simulink model "ProblemStatement1_Modulation"  (R2021a)
settings: Solver=VariableStepAuto  StartTime=0.0  StopTime=10.0  RelTol=1e-3
settings Model: Creator=psadh  LastModifiedBy=psadh

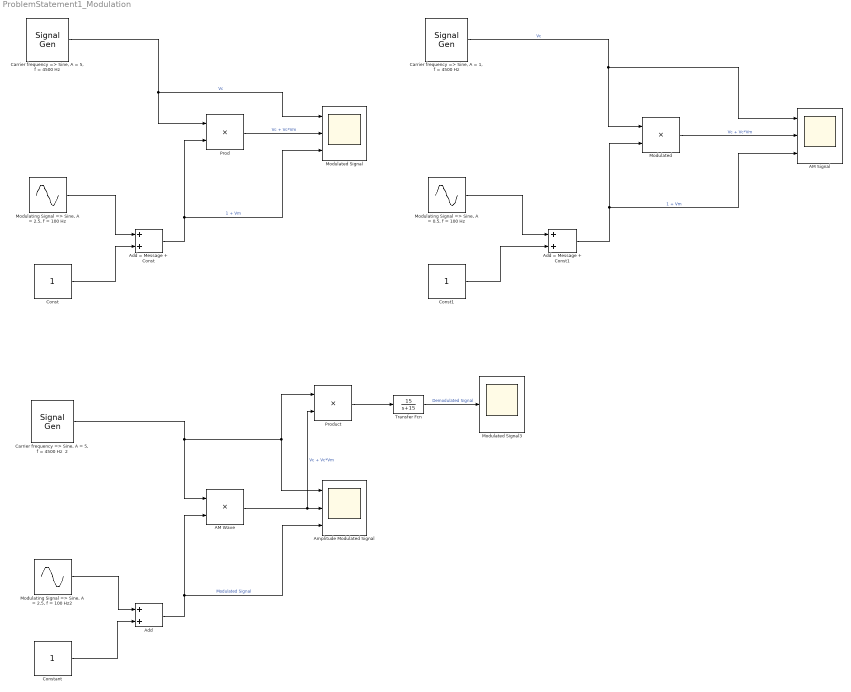
== system ProblemStatement1_Modulation ==
  AM Signal : Scope  NumInputPorts=3
  AM Wave : Product
  Add : Sum
  Add = Message + Const : Sum
  Add = Message + Const1 : Sum
  Amplitude Modulated Signal : Scope  NumInputPorts=3
  "Carrier frequency => Sine, A = 1, f = 4500 Hz  " : SignalGenerator  Frequency=2*pi*4500  Units=rad/sec
  "Carrier frequency => Sine, A = 5, f = 4500 Hz  " : SignalGenerator  Amplitude=5  Frequency=2*pi*4500  Units=rad/sec
  "Carrier frequency => Sine, A = 5, f = 4500 Hz  2" : SignalGenerator  Amplitude=5  Frequency=2*pi*4500  Units=rad/sec
  Const : Constant
  Const1 : Constant
  Constant : Constant
  "Modulated " : Product
  Modulated Signal : Scope  NumInputPorts=3
  Modulated Signal3 : Scope
  "Modulating Signal => Sine, A = 0.5, f = 100 Hz" : Sin  Amplitude=0.5  Frequency=2*pi*100  SampleTime=0
  "Modulating Signal => Sine, A = 2.5, f = 100 Hz" : Sin  Amplitude=2.5  Frequency=2*pi*100  SampleTime=0
  "Modulating Signal => Sine, A = 2.5, f = 100 Hz2" : Sin  Amplitude=2.5  Frequency=2*pi*100  SampleTime=0
  Prod : Product
  Product : Product
  Transfer Fcn : TransferFcn  Numerator=[15]  Denominator=[1 15]
  wires:
  "Modulating Signal => Sine, A = 2.5, f = 100 Hz"/1 -> Add = Message + Const/1
  Const/1 -> Add = Message + Const/2
  "Carrier frequency => Sine, A = 5, f = 4500 Hz  "/1 -> Modulated Signal/1, Prod/1  "Vc"
  Add = Message + Const/1 -> Modulated Signal/3, Prod/2  "1 + Vm"
  Prod/1 -> Modulated Signal/2  "Vc + Vc*Vm"
  "Modulated "/1 -> AM Signal/2  "Vc + Vc*Vm"
  "Carrier frequency => Sine, A = 1, f = 4500 Hz  "/1 -> AM Signal/1, "Modulated "/1  "Vc"
  Add = Message + Const1/1 -> AM Signal/3, "Modulated "/2  "1 + Vm"
  "Modulating Signal => Sine, A = 0.5, f = 100 Hz"/1 -> Add = Message + Const1/1
  Const1/1 -> Add = Message + Const1/2
  "Carrier frequency => Sine, A = 5, f = 4500 Hz  2"/1 -> Amplitude Modulated Signal/1, Product/1, AM Wave/1
  Add/1 -> Amplitude Modulated Signal/3, AM Wave/2  "Modulated Signal"
  "Modulating Signal => Sine, A = 2.5, f = 100 Hz2"/1 -> Add/1
  Constant/1 -> Add/2
  AM Wave/1 -> Product/2, Amplitude Modulated Signal/2  "Vc + Vc*Vm"
  Product/1 -> Transfer Fcn/1
  Transfer Fcn/1 -> Modulated Signal3/1  "Demodulated Signal"
